simulink library "VIS_LIB"  (Simulink 8.6)
settings: Solver=ode45  StartTime=0.0  StopTime=10.0  RelTol=1e-3
undefined symbols (not defined in the file): AC, SIXOSEM_F_WD_AC_MASTER
libraries: cdsFilt x376, cdsEpicsOut x253, cdsEpicsIn x179, cdsTP x123, VIS_LIB x95, cdsMuxMatrix x91, cdsEpicsStringIn x75, cdsFiltCtrl x72, cdsFunctionCall x70, cdsRms x59, KAGRA_UTIL x25, STATE_BIO_MASTER x5
(part 28 of 38)

== system VIS_LIB/MODAL/MODE_PARAMS/MEAS_DATE ==
  DAY : cdsEpicsIn/Subsystem  Tag=cdsEpicsIn  Description=|
      | Purpose:                                                                              
      | Create an EPICS input channel connection to the FE realtime controls.                 
      |                                                                                       
      | Operation:                                                                            
      | Outputs value from an EPICS ai record. Value is floating point with a precision of 3..
      |                                                                                       
      | Usage:                                                                                
      | Name the part with the desired EPICS channel name.
      settings: AttributesFormatString=%<Tag>
  MON : cdsEpicsIn/Subsystem  Tag=cdsEpicsIn  Description=|
      | Purpose:                                                                              
      | Create an EPICS input channel connection to the FE realtime controls.                 
      |                                                                                       
      | Operation:                                                                            
      | Outputs value from an EPICS ai record. Value is floating point with a precision of 3..
      |                                                                                       
      | Usage:                                                                                
      | Name the part with the desired EPICS channel name.
      settings: AttributesFormatString=%<Tag>
  Terminator3 : Terminator
  Terminator4 : Terminator
  Terminator5 : Terminator
  YEAR : cdsEpicsIn/Subsystem  Tag=cdsEpicsIn  Description=|
      | Purpose:                                                                              
      | Create an EPICS input channel connection to the FE realtime controls.                 
      |                                                                                       
      | Operation:                                                                            
      | Outputs value from an EPICS ai record. Value is floating point with a precision of 3..
      |                                                                                       
      | Usage:                                                                                
      | Name the part with the desired EPICS channel name.
      settings: AttributesFormatString=%<Tag>
  wires:
  DAY/1 -> Terminator3/1
  MON/1 -> Terminator4/1
  YEAR/1 -> Terminator5/1

== system VIS_LIB/MODAL/MODE_PARAMS/MN ==
  CP_COEF : Subsystem
  REL_PHASE : Subsystem

== system VIS_LIB/MODAL/MODE_PARAMS/REL_PHASE ==
  BF : cdsEpicsIn/Subsystem  Tag=cdsEpicsIn  Description=|
      | Purpose:                                                                              
      | Create an EPICS input channel connection to the FE realtime controls.                 
      |                                                                                       
      | Operation:                                                                            
      | Outputs value from an EPICS ai record. Value is floating point with a precision of 3..
      |                                                                                       
      | Usage:                                                                                
      | Name the part with the desired EPICS channel name.
      settings: AttributesFormatString=%<Tag>
  IM : cdsEpicsIn/Subsystem  Tag=cdsEpicsIn  Description=|
      | Purpose:                                                                              
      | Create an EPICS input channel connection to the FE realtime controls.                 
      |                                                                                       
      | Operation:                                                                            
      | Outputs value from an EPICS ai record. Value is floating point with a precision of 3..
      |                                                                                       
      | Usage:                                                                                
      | Name the part with the desired EPICS channel name.
      settings: AttributesFormatString=%<Tag>
  IP : cdsEpicsIn/Subsystem  Tag=cdsEpicsIn  Description=|
      | Purpose:                                                                              
      | Create an EPICS input channel connection to the FE realtime controls.                 
      |                                                                                       
      | Operation:                                                                            
      | Outputs value from an EPICS ai record. Value is floating point with a precision of 3..
      |                                                                                       
      | Usage:                                                                                
      | Name the part with the desired EPICS channel name.
      settings: AttributesFormatString=%<Tag>
  MN : cdsEpicsIn/Subsystem  Tag=cdsEpicsIn  Description=|
      | Purpose:                                                                              
      | Create an EPICS input channel connection to the FE realtime controls.                 
      |                                                                                       
      | Operation:                                                                            
      | Outputs value from an EPICS ai record. Value is floating point with a precision of 3..
      |                                                                                       
      | Usage:                                                                                
      | Name the part with the desired EPICS channel name.
      settings: AttributesFormatString=%<Tag>
  TM : cdsEpicsIn/Subsystem  Tag=cdsEpicsIn  Description=|
      | Purpose:                                                                              
      | Create an EPICS input channel connection to the FE realtime controls.                 
      |                                                                                       
      | Operation:                                                                            
      | Outputs value from an EPICS ai record. Value is floating point with a precision of 3..
      |                                                                                       
      | Usage:                                                                                
      | Name the part with the desired EPICS channel name.
      settings: AttributesFormatString=%<Tag>
  Terminator{1..5} (5 alike) : Terminator
  wires:
  MN/1 -> Terminator5/1
  TM/1 -> Terminator2/1
  BF/1 -> Terminator4/1
  IM/1 -> Terminator1/1
  IP/1 -> Terminator3/1

== system VIS_LIB/MODAL/MODE_PARAMS/TM ==
  CP_COEF : Subsystem
  REL_PHASE : Subsystem

== system VIS_LIB/MODAL/MODE_PARAMS1/MEAS_DATE ==
  DAY : cdsEpicsIn/Subsystem  Tag=cdsEpicsIn  Description=|
      | Purpose:                                                                              
      | Create an EPICS input channel connection to the FE realtime controls.                 
      |                                                                                       
      | Operation:                                                                            
      | Outputs value from an EPICS ai record. Value is floating point with a precision of 3..
      |                                                                                       
      | Usage:                                                                                
      | Name the part with the desired EPICS channel name.
      settings: AttributesFormatString=%<Tag>
  MON : cdsEpicsIn/Subsystem  Tag=cdsEpicsIn  Description=|
      | Purpose:                                                                              
      | Create an EPICS input channel connection to the FE realtime controls.                 
      |                                                                                       
      | Operation:                                                                            
      | Outputs value from an EPICS ai record. Value is floating point with a precision of 3..
      |                                                                                       
      | Usage:                                                                                
      | Name the part with the desired EPICS channel name.
      settings: AttributesFormatString=%<Tag>
  Terminator3 : Terminator
  Terminator4 : Terminator
  Terminator5 : Terminator
  YEAR : cdsEpicsIn/Subsystem  Tag=cdsEpicsIn  Description=|
      | Purpose:                                                                              
      | Create an EPICS input channel connection to the FE realtime controls.                 
      |                                                                                       
      | Operation:                                                                            
      | Outputs value from an EPICS ai record. Value is floating point with a precision of 3..
      |                                                                                       
      | Usage:                                                                                
      | Name the part with the desired EPICS channel name.
      settings: AttributesFormatString=%<Tag>
  wires:
  DAY/1 -> Terminator3/1
  MON/1 -> Terminator4/1
  YEAR/1 -> Terminator5/1

== system VIS_LIB/MODAL/MODE_PARAMS1/SENSMAT ==
  Demux : Demux  Outputs=6
  Demux1 : Demux  Outputs=6
  Ground{1..10} (10 alike) : Ground
  Mux : Mux  Inputs=5
  Mux1 : Mux  Inputs=5
  PHASE : cdsMuxMatrix/Subsystem  Tag=cdsMuxMatrix  Description=Any size matrix. Inputs and outputs must be connected using Mux and Demux parts.
      settings: AttributesFormatString=%<Tag>
  RATIO : cdsMuxMatrix/Subsystem  Tag=cdsMuxMatrix  Description=Any size matrix. Inputs and outputs must be connected using Mux and Demux parts.
      settings: AttributesFormatString=%<Tag>
  Terminator{,1..2,5..11,13..14} (12 alike) : Terminator
  wires:
  Ground5/1 -> Mux/1
  RATIO/1 -> Demux/1
  Demux/1 -> Terminator/1
  Demux1/2 -> Terminator6/1
  Demux/5 -> Terminator13/1
  Mux/1 -> RATIO/1
  Demux/3 -> Terminator10/1
  Demux1/4 -> Terminator8/1
  Mux1/1 -> PHASE/1
  Demux/2 -> Terminator9/1
  Demux1/3 -> Terminator7/1
  Demux1/1 -> Terminator5/1
  Ground4/1 -> Mux1/1
  Demux/4 -> Terminator11/1
  Demux1/5 -> Terminator14/1
  PHASE/1 -> Demux1/1
  Ground1/1 -> Mux/2
  Ground3/1 -> Mux/3
  Ground2/1 -> Mux/4
  Ground6/1 -> Mux/5
  Ground7/1 -> Mux1/2
  Ground8/1 -> Mux1/3
  Ground9/1 -> Mux1/4
  Ground10/1 -> Mux1/5
  Demux/6 -> Terminator1/1
  Demux1/6 -> Terminator2/1

== system VIS_LIB/MODAL/MODE_PARAMS1/STAGE_MOTION ==
  Demux : Demux  Outputs=5
  Demux1 : Demux  Outputs=5
  Ground1 : Ground
  Ground4 : Ground
  Mux : Mux  Inputs=1
  Mux1 : Mux  Inputs=1
  PHASE : cdsMuxMatrix/Subsystem  Tag=cdsMuxMatrix  Description=Any size matrix. Inputs and outputs must be connected using Mux and Demux parts.
      settings: AttributesFormatString=%<Tag>
  RATIO : cdsMuxMatrix/Subsystem  Tag=cdsMuxMatrix  Description=Any size matrix. Inputs and outputs must be connected using Mux and Demux parts.
      settings: AttributesFormatString=%<Tag>
  Terminator{,1..9} (10 alike) : Terminator
  wires:
  Demux/1 -> Terminator/1
  Demux/5 -> Terminator8/1
  Demux/3 -> Terminator6/1
  RATIO/1 -> Demux/1
  Demux/4 -> Terminator7/1
  Demux/2 -> Terminator5/1
  Ground4/1 -> Mux/1
  Mux/1 -> RATIO/1
  Demux1/1 -> Terminator1/1
  Demux1/5 -> Terminator9/1
  Demux1/3 -> Terminator3/1
  PHASE/1 -> Demux1/1
  Demux1/4 -> Terminator4/1
  Demux1/2 -> Terminator2/1
  Ground1/1 -> Mux1/1
  Mux1/1 -> PHASE/1

== system VIS_LIB/MODAL/MODE_PARAMS1_GAS/MEAS_DATE ==
  DAY : cdsEpicsIn/Subsystem  Tag=cdsEpicsIn  Description=|
      | Purpose:                                                                              
      | Create an EPICS input channel connection to the FE realtime controls.                 
      |                                                                                       
      | Operation:                                                                            
      | Outputs value from an EPICS ai record. Value is floating point with a precision of 3..
      |                                                                                       
      | Usage:                                                                                
      | Name the part with the desired EPICS channel name.
      settings: AttributesFormatString=%<Tag>
  MON : cdsEpicsIn/Subsystem  Tag=cdsEpicsIn  Description=|
      | Purpose:                                                                              
      | Create an EPICS input channel connection to the FE realtime controls.                 
      |                                                                                       
      | Operation:                                                                            
      | Outputs value from an EPICS ai record. Value is floating point with a precision of 3..
      |                                                                                       
      | Usage:                                                                                
      | Name the part with the desired EPICS channel name.
      settings: AttributesFormatString=%<Tag>
  Terminator3 : Terminator
  Terminator4 : Terminator
  Terminator5 : Terminator
  YEAR : cdsEpicsIn/Subsystem  Tag=cdsEpicsIn  Description=|
      | Purpose:                                                                              
      | Create an EPICS input channel connection to the FE realtime controls.                 
      |                                                                                       
      | Operation:                                                                            
      | Outputs value from an EPICS ai record. Value is floating point with a precision of 3..
      |                                                                                       
      | Usage:                                                                                
      | Name the part with the desired EPICS channel name.
      settings: AttributesFormatString=%<Tag>
  wires:
  DAY/1 -> Terminator3/1
  MON/1 -> Terminator4/1
  YEAR/1 -> Terminator5/1

== system VIS_LIB/MODAL/MODE_PARAMS1_GAS/SENSMAT ==
  Demux : Demux  Outputs=2
  Demux1 : Demux  Outputs=2
  Ground1 : Ground
  Ground5 : Ground
  Mux : Mux  Inputs=1
  Mux1 : Mux  Inputs=1
  PHASE : cdsMuxMatrix/Subsystem  Tag=cdsMuxMatrix  Description=Any size matrix. Inputs and outputs must be connected using Mux and Demux parts.
      settings: AttributesFormatString=%<Tag>
  RATIO : cdsMuxMatrix/Subsystem  Tag=cdsMuxMatrix  Description=Any size matrix. Inputs and outputs must be connected using Mux and Demux parts.
      settings: AttributesFormatString=%<Tag>
  Terminator{,1..2,9} (4 alike) : Terminator
  wires:
  Ground5/1 -> Mux/1
  RATIO/1 -> Demux/1
  Demux/1 -> Terminator/1
  Mux/1 -> RATIO/1
  Demux/2 -> Terminator9/1
  Ground1/1 -> Mux1/1
  PHASE/1 -> Demux1/1
  Demux1/1 -> Terminator1/1
  Mux1/1 -> PHASE/1
  Demux1/2 -> Terminator2/1

== system VIS_LIB/MODAL/MODE_PARAMS1_GAS/STAGE_MOTION ==
  Demux : Demux  Outputs=5
  Demux1 : Demux  Outputs=5
  Ground1 : Ground
  Ground4 : Ground
  Mux : Mux  Inputs=1
  Mux1 : Mux  Inputs=1
  PHASE : cdsMuxMatrix/Subsystem  Tag=cdsMuxMatrix  Description=Any size matrix. Inputs and outputs must be connected using Mux and Demux parts.
      settings: AttributesFormatString=%<Tag>
  RATIO : cdsMuxMatrix/Subsystem  Tag=cdsMuxMatrix  Description=Any size matrix. Inputs and outputs must be connected using Mux and Demux parts.
      settings: AttributesFormatString=%<Tag>
  Terminator{,1..9} (10 alike) : Terminator
  wires:
  Demux/1 -> Terminator/1
  Demux/5 -> Terminator8/1
  Demux/3 -> Terminator6/1
  RATIO/1 -> Demux/1
  Demux/4 -> Terminator7/1
  Demux/2 -> Terminator5/1
  Ground4/1 -> Mux/1
  Mux/1 -> RATIO/1
  Demux1/1 -> Terminator1/1
  Demux1/5 -> Terminator9/1
  Demux1/3 -> Terminator3/1
  PHASE/1 -> Demux1/1
  Demux1/4 -> Terminator4/1
  Demux1/2 -> Terminator2/1
  Ground1/1 -> Mux1/1
  Mux1/1 -> PHASE/1

== system VIS_LIB/MODAL/MOD_in_VISP/ISC ==
  ISCL : Inport
  ISCP : Inport  Port=2
  ISCY : Inport  Port=3
  CALLINE_MN : Inport  Port=4
  CALLINE_IM : Inport  Port=5
  CALLINE_TM : Inport  Port=6
  OLL : Inport  Port=7
  OLP : Inport  Port=8
  OLY : Inport  Port=9
  MNOLL : Inport  Port=10
  MNOLP : Inport  Port=11
  MNOLY : Inport  Port=12
  COM1 : VIS_LIB/UTILs/FBs_3DOF
  COM2 : VIS_LIB/UTILs/FBs_3DOF
  COM3 : VIS_LIB/UTILs/FBs_3DOF
  DRIVEALIGN : Subsystem
  FB : Subsystem
  IM : VIS_LIB/UTILs/FBs_3DOF
  MN : VIS_LIB/UTILs/FBs_3DOF
  MNOL : VIS_LIB/UTILs/FBs_3DOF
  MNOL_HP : VIS_LIB/UTILs/FBs_3DOF
  OL : VIS_LIB/UTILs/FBs_3DOF
  Sum{,1..8} (9 alike) : Sum  Inputs=++|
  TM : VIS_LIB/UTILs/FBs_3DOF
  WD : Subsystem
  MNL : Outport
  MNP : Outport  Port=2
  MNY : Outport  Port=3
  IML : Outport  Port=4
  IMP : Outport  Port=5
  IMY : Outport  Port=6
  TML : Outport  Port=7
  TMP : Outport  Port=8
  TMY : Outport  Port=9
  CAL_MN : Outport  Port=10
  CAL_IM : Outport  Port=11
  CAL_TM : Outport  Port=12
  COM3L : Outport  Port=13
  COM3P : Outport  Port=14
  COM3Y : Outport  Port=15
  wires:
  WD/3(MNYAW) -> FB/3(MNYi)
  WD/2(MNPIT) -> FB/2(MNPi)
  WD/1(MNLEN) -> FB/1(MNLi)
  WD/6(IMYAW) -> FB/6(IMYi)
  WD/5(IMPIT) -> FB/5(IMPi)
  WD/4(IMLEN) -> FB/4(IMLi)
  WD/9(TMYAW) -> FB/9(TMYi)
  WD/8(T<PIT) -> FB/8(TMPi)
  WD/7(TMLEN) -> FB/7(TMLi)
  FB/9(TMY) -> DRIVEALIGN/9(TMYi)
  FB/8(TMP) -> DRIVEALIGN/8(TMPi)
  FB/6(IMY) -> DRIVEALIGN/6(IMYi)
  FB/5(IMP) -> DRIVEALIGN/5(IMPi)
  FB/3(MNY) -> DRIVEALIGN/3(MNYi)
  FB/2(MNP) -> DRIVEALIGN/2(MNPi)
  DRIVEALIGN/9(TMY) -> TMY/1
  DRIVEALIGN/7(TML) -> TML/1
  DRIVEALIGN/8(TMP) -> TMP/1
  FB/7(TML) -> DRIVEALIGN/7(TMLi), CAL_TM/1
  DRIVEALIGN/6(IMY) -> IMY/1
  DRIVEALIGN/4(IML) -> IML/1
  DRIVEALIGN/5(IMP) -> IMP/1
  FB/4(IML) -> DRIVEALIGN/4(IMLi), CAL_IM/1
  DRIVEALIGN/3(MNY) -> MNY/1
  DRIVEALIGN/1(MNL) -> MNL/1
  DRIVEALIGN/2(MNP) -> MNP/1
  FB/1(MNL) -> DRIVEALIGN/1(MNLi), CAL_MN/1
  CALLINE_TM/1 -> Sum2/1
  CALLINE_IM/1 -> Sum1/1
  CALLINE_MN/1 -> Sum/1
  COM2/3 -> COM3/3, IM/3
  COM2/2 -> COM3/2, IM/2
  COM2/1 -> COM3/1, IM/1
  COM1/3 -> TM/3, COM2/3
  COM1/2 -> TM/2, COM2/2
  COM1/1 -> TM/1, COM2/1
  IM/1 -> Sum1/2
  TM/1 -> Sum2/2
  COM3/1 -> MN/1
  COM3/2 -> MN/2
  COM3/3 -> MN/3
  Sum/1 -> WD/1(MNL)
  Sum1/1 -> WD/4(IML)
  IM/2 -> WD/5(IMP)
  IM/3 -> WD/6(IMY)
  Sum2/1 -> WD/7(TML)
  TM/2 -> WD/8(TMP)
  TM/3 -> WD/9(TMY)
  ISCL/1 -> Sum3/2
  Sum3/1 -> COM1/1
  ISCP/1 -> Sum4/2
  Sum4/1 -> COM1/2
  Sum5/1 -> COM1/3
  ISCY/1 -> Sum5/2
  OL/3 -> Sum5/1
  OL/2 -> Sum4/1
  OL/1 -> Sum3/1
  OLL/1 -> OL/1
  OLP/1 -> OL/2
  OLY/1 -> OL/3
  Sum6/1 -> MNOL/1
  Sum7/1 -> MNOL/2
  Sum8/1 -> MNOL/3
  MNOL/1 -> COM3L/1, Sum/2
  MN/1 -> Sum6/2
  MN/2 -> Sum7/2
  MN/3 -> Sum8/2
  MNOL/2 -> WD/2(MNP), COM3P/1
  MNOL/3 -> WD/3(MNY), COM3Y/1
  MNOLL/1 -> MNOL_HP/1
  MNOLP/1 -> MNOL_HP/2
  MNOLY/1 -> MNOL_HP/3
  MNOL_HP/3 -> Sum8/1
  MNOL_HP/2 -> Sum7/1
  MNOL_HP/1 -> Sum6/1

== system VIS_LIB/MODAL/MOD_in_VISP/Sum ==
  MNL1 : Inport
  MNT1 : Inport  Port=2
  MNV1 : Inport  Port=3
  MNR1 : Inport  Port=4
  MNP1 : Inport  Port=5
  MNY1 : Inport  Port=6
  IML1 : Inport  Port=7
  IMT1 : Inport  Port=8
  IMV1 : Inport  Port=9
  IMR1 : Inport  Port=10
  IMP1 : Inport  Port=11
  IMY1 : Inport  Port=12
  TML1 : Inport  Port=13
  TMP1 : Inport  Port=14
  TMY1 : Inport  Port=15
  MNL2 : Inport  Port=16
  MNP2 : Inport  Port=17
  MNY2 : Inport  Port=18
  IML2 : Inport  Port=19
  IMP2 : Inport  Port=20
  IMY2 : Inport  Port=21
  TML2 : Inport  Port=22
  TMP2 : Inport  Port=23
  TMY2 : Inport  Port=24
  Ground{1..6} (6 alike) : Ground
  sum{10..24} (15 alike) : VIS_LIB/MODAL/sum1
  MNL : Outport
  MNT : Outport  Port=2
  MNV : Outport  Port=3
  MNR : Outport  Port=4
  MNP : Outport  Port=5
  MNY : Outport  Port=6
  IML : Outport  Port=7
  IMT : Outport  Port=8
  IMV : Outport  Port=9
  IMR : Outport  Port=10
  IMP : Outport  Port=11
  IMY : Outport  Port=12
  TML : Outport  Port=13
  TMP : Outport  Port=14
  TMY : Outport  Port=15
  wires:
  Ground6/1 -> sum17/2
  Ground5/1 -> sum18/2
  TMY2/1 -> sum24/2
  TMP2/1 -> sum23/2
  TML2/1 -> sum22/2
  IMY2/1 -> sum21/2
  IMP2/1 -> sum20/2
  Ground4/1 -> sum19/2
  IML2/1 -> sum16/2
  MNY2/1 -> sum15/2
  MNP2/1 -> sum14/2
  Ground3/1 -> sum13/2
  Ground1/1 -> sum12/2
  Ground2/1 -> sum11/2
  MNL2/1 -> sum10/2
  TMY1/1 -> sum24/1
  sum24/1 -> TMY/1
  TMP1/1 -> sum23/1
  sum23/1 -> TMP/1
  TML1/1 -> sum22/1
  sum22/1 -> TML/1
  IMY1/1 -> sum21/1
  sum21/1 -> IMY/1
  IMP1/1 -> sum20/1
  sum20/1 -> IMP/1
  IMR1/1 -> sum19/1
  sum19/1 -> IMR/1
  IMV1/1 -> sum18/1
  sum18/1 -> IMV/1
  IMT1/1 -> sum17/1
  sum17/1 -> IMT/1
  IML1/1 -> sum16/1
  sum16/1 -> IML/1
  MNY1/1 -> sum15/1
  sum15/1 -> MNY/1
  MNP1/1 -> sum14/1
  sum14/1 -> MNP/1
  MNR1/1 -> sum13/1
  sum13/1 -> MNR/1
  MNV1/1 -> sum12/1
  sum12/1 -> MNV/1
  MNT1/1 -> sum11/1
  sum11/1 -> MNT/1
  MNL1/1 -> sum10/1
  sum10/1 -> MNL/1

== system VIS_LIB/MODAL/MOD_in_VIST/ISC_WD ==
  L : Inport
  P : Inport  Port=2
  Y : Inport  Port=3
  BFL_RMS : cdsRms/Subsystem  Tag=cdsRms  Description=|
      | Purpose:
      | Calculate an RMS based on the input signal.
      settings: AttributesFormatString=%<Tag>
  BFP_RMS : cdsRms/Subsystem  Tag=cdsRms  Description=|
      | Purpose:
      | Calculate an RMS based on the input signal.
      settings: AttributesFormatString=%<Tag>
  BFY_RMS1 : cdsRms/Subsystem  Tag=cdsRms  Description=|
      | Purpose:
      | Calculate an RMS based on the input signal.
      settings: AttributesFormatString=%<Tag>
  BF_LEN : KAGRA_UTIL/RAMPHOLD
  BF_PIT : KAGRA_UTIL/RAMPHOLD
  BF_YAW : KAGRA_UTIL/RAMPHOLD
  BP_BF_LEN : cdsFilt/Subsystem  Tag=cdsFilt  Description=|
      | Purpose:                                                                                                                                                                                                                                  
      | Standard CDS IIR filter module.                                                                                                                                                                                                           
      |                                                                                                                                                                                                                                           
      | Operation:                                                                                                                                                                                                                                
      | Consists of 10 second order section IIR filters, plus a ramped gain stage. In FE code, also provides pre-defined test points and excitation channel inputs. The filter coefficients are defined in the LIGO system using the 'foton' tool.
      |                                                                                                                                                                                                                                           
      | Usage:                                                                                                                                                                                                                                    
      | Name the part with the desired filter module name.
      settings: AttributesFormatString=%<Tag>
  BP_BF_PIT : cdsFilt/Subsystem  Tag=cdsFilt  Description=|
      | Purpose:                                                                                                                                                                                                                                  
      | Standard CDS IIR filter module.                                                                                                                                                                                                           
      |                                                                                                                                                                                                                                           
      | Operation:                                                                                                                                                                                                                                
      | Consists of 10 second order section IIR filters, plus a ramped gain stage. In FE code, also provides pre-defined test points and excitation channel inputs. The filter coefficients are defined in the LIGO system using the 'foton' tool.
      |                                                                                                                                                                                                                                           
      | Usage:                                                                                                                                                                                                                                    
      | Name the part with the desired filter module name.
      settings: AttributesFormatString=%<Tag>
  BP_BF_YAW : cdsFilt/Subsystem  Tag=cdsFilt  Description=|
      | Purpose:                                                                                                                                                                                                                                  
      | Standard CDS IIR filter module.                                                                                                                                                                                                           
      |                                                                                                                                                                                                                                           
      | Operation:                                                                                                                                                                                                                                
      | Consists of 10 second order section IIR filters, plus a ramped gain stage. In FE code, also provides pre-defined test points and excitation channel inputs. The filter coefficients are defined in the LIGO system using the 'foton' tool.
      |                                                                                                                                                                                                                                           
      | Usage:                                                                                                                                                                                                                                    
      | Name the part with the desired filter module name.
      settings: AttributesFormatString=%<Tag>
  Operator1 : RelationalOperator  Operator=>  OutDataTypeStr=boolean
  Operator2 : RelationalOperator  Operator=>  OutDataTypeStr=boolean
  Operator3 : RelationalOperator  Operator=>  OutDataTypeStr=boolean
  RMS_BF_LEN : cdsEpicsOut/Subsystem  Tag=cdsEpicsOutput  Description=|
      | Purpose:                                          
      | Output a FE signal to an EPICS channel.           
      |                                                   
      | Operation:                                        
      | Takes input value and passes it to EPICS record.  
      |                                                   
      | Usage:                                            
      | Name the part with the desired EPICS rrecord name.
      settings: AttributesFormatString=%<Tag>
  RMS_BF_PIT : cdsEpicsOut/Subsystem  Tag=cdsEpicsOutput  Description=|
      | Purpose:                                          
      | Output a FE signal to an EPICS channel.           
      |                                                   
      | Operation:                                        
      | Takes input value and passes it to EPICS record.  
      |                                                   
      | Usage:                                            
      | Name the part with the desired EPICS rrecord name.
      settings: AttributesFormatString=%<Tag>
  RMS_BF_YAW : cdsEpicsOut/Subsystem  Tag=cdsEpicsOutput  Description=|
      | Purpose:                                          
      | Output a FE signal to an EPICS channel.           
      |                                                   
      | Operation:                                        
      | Takes input value and passes it to EPICS record.  
      |                                                   
      | Usage:                                            
      | Name the part with the desired EPICS rrecord name.
      settings: AttributesFormatString=%<Tag>
  RMS_THR_BF_LEN : cdsEpicsIn/Subsystem  Tag=cdsEpicsIn  Description=|
      | Purpose:                                                                              
      | Create an EPICS input channel connection to the FE realtime controls.                 
      |                                                                                       
      | Operation:                                                                            
      | Outputs value from an EPICS ai record. Value is floating point with a precision of 3..
      |                                                                                       
      | Usage:                                                                                
      | Name the part with the desired EPICS channel name.
      settings: AttributesFormatString=%<Tag>
  RMS_THR_BF_PIT : cdsEpicsIn/Subsystem  Tag=cdsEpicsIn  Description=|
      | Purpose:                                                                              
      | Create an EPICS input channel connection to the FE realtime controls.                 
      |                                                                                       
      | Operation:                                                                            
      | Outputs value from an EPICS ai record. Value is floating point with a precision of 3..
      |                                                                                       
      | Usage:                                                                                
      | Name the part with the desired EPICS channel name.
      settings: AttributesFormatString=%<Tag>
  RMS_THR_BF_YAW : cdsEpicsIn/Subsystem  Tag=cdsEpicsIn  Description=|
      | Purpose:                                                                              
      | Create an EPICS input channel connection to the FE realtime controls.                 
      |                                                                                       
      | Operation:                                                                            
      | Outputs value from an EPICS ai record. Value is floating point with a precision of 3..
      |                                                                                       
      | Usage:                                                                                
      | Name the part with the desired EPICS channel name.
      settings: AttributesFormatString=%<Tag>
  LEN : Outport
  PIT : Outport  Port=2
  YAW : Outport  Port=3
  wires:
  BP_BF_LEN/1 -> BFL_RMS/1
  RMS_BF_LEN/1 -> Operator1/1
  L/1 -> BF_LEN/1, BP_BF_LEN/1
  RMS_THR_BF_LEN/1 -> Operator1/2
  BFL_RMS/1 -> RMS_BF_LEN/1
  BP_BF_PIT/1 -> BFP_RMS/1
  RMS_BF_PIT/1 -> Operator2/1
  RMS_THR_BF_PIT/1 -> Operator2/2
  BFP_RMS/1 -> RMS_BF_PIT/1
  BP_BF_YAW/1 -> BFY_RMS1/1
  RMS_BF_YAW/1 -> Operator3/1
  Y/1 -> BF_YAW/1, BP_BF_YAW/1
  RMS_THR_BF_YAW/1 -> Operator3/2
  BFY_RMS1/1 -> RMS_BF_YAW/1
  Operator1/1 -> BF_LEN/2
  BF_LEN/1 -> LEN/1
  P/1 -> BF_PIT/1, BP_BF_PIT/1
  Operator2/1 -> BF_PIT/2
  BF_PIT/1 -> PIT/1
  Operator3/1 -> BF_YAW/2
  BF_YAW/1 -> YAW/1

== system VIS_LIB/MODAL/SENSDIAG/BF ==
  AMP : cdsMuxMatrix/Subsystem  Tag=cdsMuxMatrix  Description=Any size matrix. Inputs and outputs must be connected using Mux and Demux parts.
      settings: AttributesFormatString=%<Tag>
  Demux1 : Demux  Outputs=6
  Demux2 : Demux  Outputs=6
  Ground{,1..11} (12 alike) : Ground
  MODEINDEX : Subsystem
  Mux : Mux  Inputs=6
  Mux1 : Mux  Inputs=6
  PHASE : cdsMuxMatrix/Subsystem  Tag=cdsMuxMatrix  Description=Any size matrix. Inputs and outputs must be connected using Mux and Demux parts.
      settings: AttributesFormatString=%<Tag>
  Terminator{,1..11} (12 alike) : Terminator
  wires:
  Mux/1 -> AMP/1
  AMP/1 -> Demux2/1
  Ground/1 -> Mux/1
  Demux2/1 -> Terminator/1
  Demux2/2 -> Terminator1/1
  Demux2/3 -> Terminator2/1
  Demux2/4 -> Terminator3/1
  Demux2/5 -> Terminator4/1
  Demux2/6 -> Terminator5/1
  Ground1/1 -> Mux/2
  Ground2/1 -> Mux/3
  Ground3/1 -> Mux/4
  Ground4/1 -> Mux/5
  Ground5/1 -> Mux/6
  Mux1/1 -> PHASE/1
  PHASE/1 -> Demux1/1
  Ground6/1 -> Mux1/1
  Demux1/1 -> Terminator6/1
  Demux1/2 -> Terminator7/1
  Demux1/3 -> Terminator8/1
  Demux1/4 -> Terminator9/1
  Demux1/5 -> Terminator10/1
  Demux1/6 -> Terminator11/1
  Ground7/1 -> Mux1/2
  Ground8/1 -> Mux1/3
  Ground9/1 -> Mux1/4
  Ground10/1 -> Mux1/5
  Ground11/1 -> Mux1/6

== system VIS_LIB/MODAL/SENSDIAG/GAS ==
  Demux1 : Demux  Outputs=5
  Demux2 : Demux  Outputs=5
  Ground{,1..4,6..10} (10 alike) : Ground
  MODEINDEX : Subsystem
  Mux : Mux  Inputs=5
  Mux1 : Mux  Inputs=5
  PHASE : cdsMuxMatrix/Subsystem  Tag=cdsMuxMatrix  Description=Any size matrix. Inputs and outputs must be connected using Mux and Demux parts.
      settings: AttributesFormatString=%<Tag>
  RATIO : cdsMuxMatrix/Subsystem  Tag=cdsMuxMatrix  Description=Any size matrix. Inputs and outputs must be connected using Mux and Demux parts.
      settings: AttributesFormatString=%<Tag>
  Terminator{,1..4,6..10} (10 alike) : Terminator
  wires:
  Mux/1 -> RATIO/1
  RATIO/1 -> Demux2/1
  Ground/1 -> Mux/1
  Demux2/1 -> Terminator/1
  Demux2/2 -> Terminator1/1
  Demux2/3 -> Terminator2/1
  Demux2/4 -> Terminator3/1
  Demux2/5 -> Terminator4/1
  Ground1/1 -> Mux/2
  Ground2/1 -> Mux/3
  Ground3/1 -> Mux/4
  Ground4/1 -> Mux/5
  Mux1/1 -> PHASE/1
  PHASE/1 -> Demux1/1
  Ground6/1 -> Mux1/1
  Demux1/1 -> Terminator6/1
  Demux1/2 -> Terminator7/1
  Demux1/3 -> Terminator8/1
  Demux1/4 -> Terminator9/1
  Demux1/5 -> Terminator10/1
  Ground7/1 -> Mux1/2
  Ground8/1 -> Mux1/3
  Ground9/1 -> Mux1/4
  Ground10/1 -> Mux1/5

== system VIS_LIB/MODAL/SENSDIAG/IM ==
  AMP : cdsMuxMatrix/Subsystem  Tag=cdsMuxMatrix  Description=Any size matrix. Inputs and outputs must be connected using Mux and Demux parts.
      settings: AttributesFormatString=%<Tag>
  Demux1 : Demux  Outputs=6
  Demux2 : Demux  Outputs=6
  Ground{,1..11} (12 alike) : Ground
  MODEINDEX : Subsystem
  Mux : Mux  Inputs=6
  Mux1 : Mux  Inputs=6
  PHASE : cdsMuxMatrix/Subsystem  Tag=cdsMuxMatrix  Description=Any size matrix. Inputs and outputs must be connected using Mux and Demux parts.
      settings: AttributesFormatString=%<Tag>
  Terminator{,1..11} (12 alike) : Terminator
  wires:
  Mux/1 -> AMP/1
  AMP/1 -> Demux2/1
  Ground/1 -> Mux/1
  Demux2/1 -> Terminator/1
  Demux2/2 -> Terminator1/1
  Demux2/3 -> Terminator2/1
  Demux2/4 -> Terminator3/1
  Demux2/5 -> Terminator4/1
  Demux2/6 -> Terminator5/1
  Ground1/1 -> Mux/2
  Ground2/1 -> Mux/3
  Ground3/1 -> Mux/4
  Ground4/1 -> Mux/5
  Ground5/1 -> Mux/6
  Mux1/1 -> PHASE/1
  PHASE/1 -> Demux1/1
  Ground6/1 -> Mux1/1
  Demux1/1 -> Terminator6/1
  Demux1/2 -> Terminator7/1
  Demux1/3 -> Terminator8/1
  Demux1/4 -> Terminator9/1
  Demux1/5 -> Terminator10/1
  Demux1/6 -> Terminator11/1
  Ground7/1 -> Mux1/2
  Ground8/1 -> Mux1/3
  Ground9/1 -> Mux1/4
  Ground10/1 -> Mux1/5
  Ground11/1 -> Mux1/6

== system VIS_LIB/MODAL/SENSDIAG/IP ==
  AMP : cdsMuxMatrix/Subsystem  Tag=cdsMuxMatrix  Description=Any size matrix. Inputs and outputs must be connected using Mux and Demux parts.
      settings: AttributesFormatString=%<Tag>
  Demux1 : Demux  Outputs=6
  Demux2 : Demux  Outputs=6
  Ground{,1..11} (12 alike) : Ground
  MODEINDEX : Subsystem
  Mux : Mux  Inputs=6
  Mux1 : Mux  Inputs=6
  PHASE : cdsMuxMatrix/Subsystem  Tag=cdsMuxMatrix  Description=Any size matrix. Inputs and outputs must be connected using Mux and Demux parts.
      settings: AttributesFormatString=%<Tag>
  Terminator{,1..11} (12 alike) : Terminator
  wires:
  Mux/1 -> AMP/1
  AMP/1 -> Demux2/1
  Ground/1 -> Mux/1
  Demux2/1 -> Terminator/1
  Demux2/2 -> Terminator1/1
  Demux2/3 -> Terminator2/1
  Demux2/4 -> Terminator3/1
  Demux2/5 -> Terminator4/1
  Demux2/6 -> Terminator5/1
  Ground1/1 -> Mux/2
  Ground2/1 -> Mux/3
  Ground3/1 -> Mux/4
  Ground4/1 -> Mux/5
  Ground5/1 -> Mux/6
  Mux1/1 -> PHASE/1
  PHASE/1 -> Demux1/1
  Ground6/1 -> Mux1/1
  Demux1/1 -> Terminator6/1
  Demux1/2 -> Terminator7/1
  Demux1/3 -> Terminator8/1
  Demux1/4 -> Terminator9/1
  Demux1/5 -> Terminator10/1
  Demux1/6 -> Terminator11/1
  Ground7/1 -> Mux1/2
  Ground8/1 -> Mux1/3
  Ground9/1 -> Mux1/4
  Ground10/1 -> Mux1/5
  Ground11/1 -> Mux1/6

== system VIS_LIB/MODAL/SENSDIAG/MN ==
  AMP : cdsMuxMatrix/Subsystem  Tag=cdsMuxMatrix  Description=Any size matrix. Inputs and outputs must be connected using Mux and Demux parts.
      settings: AttributesFormatString=%<Tag>
  Demux1 : Demux  Outputs=6
  Demux2 : Demux  Outputs=6
  Ground{,1..11} (12 alike) : Ground
  MODEINDEX : Subsystem
  Mux : Mux  Inputs=6
  Mux1 : Mux  Inputs=6
  PHASE : cdsMuxMatrix/Subsystem  Tag=cdsMuxMatrix  Description=Any size matrix. Inputs and outputs must be connected using Mux and Demux parts.
      settings: AttributesFormatString=%<Tag>
  Terminator{,1..11} (12 alike) : Terminator
  wires:
  Mux/1 -> AMP/1
  AMP/1 -> Demux2/1
  Ground/1 -> Mux/1
  Demux2/1 -> Terminator/1
  Demux2/2 -> Terminator1/1
  Demux2/3 -> Terminator2/1
  Demux2/4 -> Terminator3/1
  Demux2/5 -> Terminator4/1
  Demux2/6 -> Terminator5/1
  Ground1/1 -> Mux/2
  Ground2/1 -> Mux/3
  Ground3/1 -> Mux/4
  Ground4/1 -> Mux/5
  Ground5/1 -> Mux/6
  Mux1/1 -> PHASE/1
  PHASE/1 -> Demux1/1
  Ground6/1 -> Mux1/1
  Demux1/1 -> Terminator6/1
  Demux1/2 -> Terminator7/1
  Demux1/3 -> Terminator8/1
  Demux1/4 -> Terminator9/1
  Demux1/5 -> Terminator10/1
  Demux1/6 -> Terminator11/1
  Ground7/1 -> Mux1/2
  Ground8/1 -> Mux1/3
  Ground9/1 -> Mux1/4
  Ground10/1 -> Mux1/5
  Ground11/1 -> Mux1/6

== system VIS_LIB/MODAL/SENSDIAG/TM ==
  AMP : cdsMuxMatrix/Subsystem  Tag=cdsMuxMatrix  Description=Any size matrix. Inputs and outputs must be connected using Mux and Demux parts.
      settings: AttributesFormatString=%<Tag>
  Demux1 : Demux  Outputs=6
  Demux2 : Demux  Outputs=6
  Ground{,1..11} (12 alike) : Ground
  MODEINDEX : Subsystem
  Mux : Mux  Inputs=6
  Mux1 : Mux  Inputs=6
  PHASE : cdsMuxMatrix/Subsystem  Tag=cdsMuxMatrix  Description=Any size matrix. Inputs and outputs must be connected using Mux and Demux parts.
      settings: AttributesFormatString=%<Tag>
  Terminator{,1..11} (12 alike) : Terminator
  wires:
  Mux/1 -> AMP/1
  AMP/1 -> Demux2/1
  Ground/1 -> Mux/1
  Demux2/1 -> Terminator/1
  Demux2/2 -> Terminator1/1
  Demux2/3 -> Terminator2/1
  Demux2/4 -> Terminator3/1
  Demux2/5 -> Terminator4/1
  Demux2/6 -> Terminator5/1
  Ground1/1 -> Mux/2
  Ground2/1 -> Mux/3
  Ground3/1 -> Mux/4
  Ground4/1 -> Mux/5
  Ground5/1 -> Mux/6
  Mux1/1 -> PHASE/1
  PHASE/1 -> Demux1/1
  Ground6/1 -> Mux1/1
  Demux1/1 -> Terminator6/1
  Demux1/2 -> Terminator7/1
  Demux1/3 -> Terminator8/1
  Demux1/4 -> Terminator9/1
  Demux1/5 -> Terminator10/1
  Demux1/6 -> Terminator11/1
  Ground7/1 -> Mux1/2
  Ground8/1 -> Mux1/3
  Ground9/1 -> Mux1/4
  Ground10/1 -> Mux1/5
  Ground11/1 -> Mux1/6

== system VIS_LIB/MODAL/inputproc/CAL ==
  In1 : Inport
  In2 : Inport  Port=2
  In3 : Inport  Port=3
  In4 : Inport  Port=4
  In5 : Inport  Port=5
  In6 : Inport  Port=6
  In7 : Inport  Port=7
  In8 : Inport  Port=8
  In9 : Inport  Port=9
  In10 : Inport  Port=10
  In11 : Inport  Port=11
  In12 : Inport  Port=12
  In13 : Inport  Port=13
  In14 : Inport  Port=14
  In15 : Inport  Port=15
  In16 : Inport  Port=16
  In17 : Inport  Port=17
  In18 : Inport  Port=18
  In19 : Inport  Port=19
  In20 : Inport  Port=20
  In21 : Inport  Port=21
  In22 : Inport  Port=22
  In23 : Inport  Port=23
  In24 : Inport  Port=24
  In25 : Inport  Port=25
  In26 : Inport  Port=26
  In27 : Inport  Port=27
  In28 : Inport  Port=28
  In29 : Inport  Port=29
  In30 : Inport  Port=30
  In31 : Inport  Port=31
  In32 : Inport  Port=32
  In33 : Inport  Port=33
  In34 : Inport  Port=34
  In35 : Inport  Port=35
  In36 : Inport  Port=36
  BF : Subsystem
  IM : Subsystem
  IP : Subsystem
  MN : Subsystem
  MNOL : Subsystem
  TM : Subsystem
  Out1 : Outport
  Out2 : Outport  Port=2
  Out3 : Outport  Port=3
  Out4 : Outport  Port=4
  Out5 : Outport  Port=5
  Out6 : Outport  Port=6
  Out7 : Outport  Port=7
  Out8 : Outport  Port=8
  Out9 : Outport  Port=9
  Out10 : Outport  Port=10
  Out11 : Outport  Port=11
  Out12 : Outport  Port=12
  Out13 : Outport  Port=13
  Out14 : Outport  Port=14
  Out15 : Outport  Port=15
  Out16 : Outport  Port=16
  Out17 : Outport  Port=17
  Out18 : Outport  Port=18
  Out19 : Outport  Port=19
  Out20 : Outport  Port=20
  Out21 : Outport  Port=21
  Out22 : Outport  Port=22
  Out23 : Outport  Port=23
  Out24 : Outport  Port=24
  Out25 : Outport  Port=25
  Out26 : Outport  Port=26
  Out27 : Outport  Port=27
  Out28 : Outport  Port=28
  Out29 : Outport  Port=29
  Out30 : Outport  Port=30
  Out31 : Outport  Port=31
  Out32 : Outport  Port=32
  Out33 : Outport  Port=33
  Out34 : Outport  Port=34
  Out35 : Outport  Port=35
  Out36 : Outport  Port=36
  wires:
  IP/4(ROL_OUT) -> Out4/1
  IP/5(PIT_OUT) -> Out5/1
  IP/6(YAW_OUT) -> Out6/1
  In2/1 -> IP/2(TRA_IN)
  IM/4(ROL_OUT) -> Out22/1
  IM/3(VER_OUT) -> Out21/1
  IM/5(PIT_OUT) -> Out23/1
  IM/6(YAW_OUT) -> Out24/1
  In25/1 -> TM/1(LEN_IN)
  In1/1 -> IP/1(LEN_IN)
  IP/1(LEN_OUT) -> Out1/1
  IP/2(TRA_OUT) -> Out2/1
  IP/3(VER_OUT) -> Out3/1
  BF/2(TRA_OUT) -> Out8/1
  BF/3(VER_OUT) -> Out9/1
  BF/4(ROL_OUT) -> Out10/1
  BF/5(PIT_OUT) -> Out11/1
  In26/1 -> TM/2(TRA_IN)
  In27/1 -> TM/3(VER_IN)
  In28/1 -> TM/4(ROL_IN)
  In29/1 -> TM/5(PIT_IN)
  In4/1 -> IP/4(ROL_IN)
  In3/1 -> IP/3(VER_IN)
  In5/1 -> IP/5(PIT_IN)
  In6/1 -> IP/6(YAW_IN)
  In7/1 -> BF/1(LEN_IN)
  TM/6(YAW_OUT) -> Out30/1
  MN/4(ROL_OUT) -> Out16/1
  MN/5(PIT_OUT) -> Out17/1
  MN/6(YAW_OUT) -> Out18/1
  BF/1(LEN_OUT) -> Out7/1
  TM/4(ROL_OUT) -> Out28/1
  In24/1 -> IM/6(YAW_IN)
  IM/1(LEN_OUT) -> Out19/1
  MN/3(VER_OUT) -> Out15/1
  IM/2(TRA_OUT) -> Out20/1
  In18/1 -> MN/6(YAW_IN)
  In17/1 -> MN/5(PIT_IN)
  MN/1(LEN_OUT) -> Out13/1
  MN/2(TRA_OUT) -> Out14/1
  In19/1 -> IM/1(LEN_IN)
  BF/6(YAW_OUT) -> Out12/1
  In20/1 -> IM/2(TRA_IN)
  In21/1 -> IM/3(VER_IN)
  In22/1 -> IM/4(ROL_IN)
  In23/1 -> IM/5(PIT_IN)
  TM/1(LEN_OUT) -> Out25/1
  In30/1 -> TM/6(YAW_IN)
  TM/3(VER_OUT) -> Out27/1
  TM/2(TRA_OUT) -> Out26/1
  TM/5(PIT_OUT) -> Out29/1
  In8/1 -> BF/2(TRA_IN)
  In9/1 -> BF/3(VER_IN)
  In10/1 -> BF/4(ROL_IN)
  In11/1 -> BF/5(PIT_IN)
  In13/1 -> MN/1(LEN_IN)
  In12/1 -> BF/6(YAW_IN)
  In14/1 -> MN/2(TRA_IN)
  In15/1 -> MN/3(VER_IN)
  In16/1 -> MN/4(ROL_IN)
  In32/1 -> MNOL/2(TRA_IN)
  In33/1 -> MNOL/3(VER_IN)
  In34/1 -> MNOL/4(ROL_IN)
  In35/1 -> MNOL/5(PIT_IN)
  MNOL/6(YAW_OUT) -> Out36/1
  MNOL/4(ROL_OUT) -> Out34/1
  In36/1 -> MNOL/6(YAW_IN)
  MNOL/3(VER_OUT) -> Out33/1
  MNOL/2(TRA_OUT) -> Out32/1
  MNOL/5(PIT_OUT) -> Out35/1
  MNOL/1(LEN_OUT) -> Out31/1
  In31/1 -> MNOL/1(LEN_IN)
